simulink library "INT_LsComp_TrqCalc"  (R2016b)
settings: Solver=VariableStepAuto  StartTime=0.0  StopTime=10.0  RelTol=1e-3
settings Model: Creator=Administrator  LastModifiedBy=Administrator

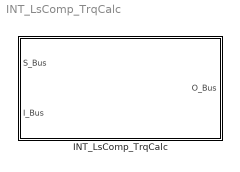
== system INT_LsComp_TrqCalc ==
  INT_LsComp_TrqCalc : Subsystem

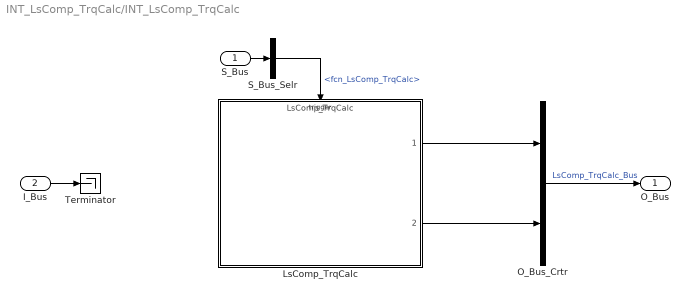
== system INT_LsComp_TrqCalc/INT_LsComp_TrqCalc ==
  S_Bus : Inport
  I_Bus : Inport  Port=2
  LsComp_TrqCalc : ModelReference  ModelNameDialog=LsComp_TrqCalc  SimulationMode=Normal  ModelReferenceVersion=1.2  TriggerPortName=function  TriggerPortTriggerType=function-call  TriggerPortStatesWhenEnabling=held
  O_Bus_Crtr : BusCreator  Inputs=2
  S_Bus_Selr : BusSelector  OutputSignals=fcn_LsComp_TrqCalc
  Terminator : Terminator
  O_Bus : Outport
  wires:
  S_Bus_Selr/1 -> LsComp_TrqCalc/Trigger  "<fcn_LsComp_TrqCalc>"
  S_Bus/1 -> S_Bus_Selr/1
  I_Bus/1 -> Terminator/1
  O_Bus_Crtr/1 -> O_Bus/1  "LsComp_TrqCalc_Bus"
  LsComp_TrqCalc/1 -> O_Bus_Crtr/1
  LsComp_TrqCalc/2 -> O_Bus_Crtr/2
